simulink model "couche_0"  (R2019b)
settings: Solver=ode23t  StartTime=0.0  StopTime=50  RelTol=1e-3
InitFcn:
  | S = 80   % m2
  | e = 30   % cm
  | p = 2500  % kg/m3
  | lamda = 1.65  %  W/(K.m)
  | C = 880  % J/kg/K
  | k_conv = 25   %  W/(m2.K)
libraries: fl_lib x12, nesl_utility x3
settings Model: Creator=Ivan  LastModifiedBy=Ivan

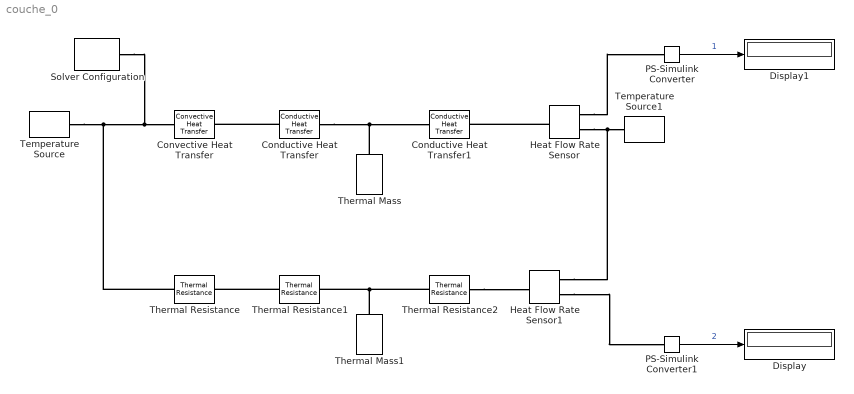
== system couche_0 ==
  Conductive Heat Transfer : fl_lib/Thermal/Thermal Elements/Conductive Heat Transfer  area=S m^2  thickness=e/2 m  th_cond=lamda W/(m*K)  T_specify=off  T_priority=None  T=0 K  T_nominal_specify=off  T_nominal_unit=K  T_nominal_value=1  Q_specify=off  Q_priority=None  Q=0 W  Q_nominal_specify=off  Q_nominal_unit=W  Q_nominal_value=1
      settings: SourceProductName=Simscape
  Conductive Heat Transfer1 : fl_lib/Thermal/Thermal Elements/Conductive Heat Transfer  area=S m^2  thickness=e/2 m  th_cond=lamda W/(m*K)  T_specify=off  T_priority=None  T=0 K  T_nominal_specify=off  T_nominal_unit=K  T_nominal_value=1  Q_specify=off  Q_priority=None  Q=0 W  Q_nominal_specify=off  Q_nominal_unit=W  Q_nominal_value=1
      settings: SourceProductName=Simscape
  Convective Heat Transfer : fl_lib/Thermal/Thermal Elements/Convective Heat Transfer  area=S m^2  heat_tr_coeff=k_conv W/(m^2 * K)  T_specify=off  T_priority=None  T=0 K  T_nominal_specify=off  T_nominal_unit=K  T_nominal_value=1  Q_specify=off  Q_priority=None  Q=0 W  Q_nominal_specify=off  Q_nominal_unit=W  Q_nominal_value=1
  Display : Display
  Display1 : Display
  Heat Flow Rate Sensor : fl_lib/Thermal/Thermal Sensors/Heat Flow Rate Sensor
      settings: SourceProductName=Simscape  SourceProductBaseCode=SS
  Heat Flow Rate Sensor1 : fl_lib/Thermal/Thermal Sensors/Heat Flow Rate Sensor
      settings: SourceProductName=Simscape  SourceProductBaseCode=SS
  PS-Simulink Converter : nesl_utility/PS-Simulink Converter  PhysicalDomain=network_engine_domain  SubClassName=ps_output  LeftPortType=input  RightPortType=output  PseudoPeriodic=off  Frequencies=[]  Unit=W  AffineConversion=off
  PS-Simulink Converter1 : nesl_utility/PS-Simulink Converter  PhysicalDomain=network_engine_domain  SubClassName=ps_output  LeftPortType=input  RightPortType=output  PseudoPeriodic=off  Frequencies=[]  Unit=W  AffineConversion=off
  Solver Configuration : nesl_utility/Solver Configuration  PhysicalDomain=network_engine_domain  SubClassName=solver  LeftPortType=input  RightPortType=generic  Tones=[]  Harmonics=[]  SimulateNoise=off  Profile=off  UseLocalSampling=off  EnableSwitchedLinearOptims=on  FrequencyDomain=off  UseCCode=off  RelTol=0.001  AbsTol=1e-06  MinStep=1e-09  ToWorkspace=off  RevertToSquareIcSolve=off  NumHomotopyIterations=100  PhasorMode=off  PhasorModeNumHarmonics=1  DoDC=off  ResidualTolerance=1e-09  UseLocalSolver=off  LocalSolverChoice=NE_BACKWARD_EULER_ADVANCER  LocalSolverSampleTime=0.001  DoFixedCost=off  MaxNonlinIter=3  MaxModeIter=2  LinearAlgebra=auto  EquationFormulation=NE_TIME_EF  DelaysMemoryBudget=1024  AutomaticFiltering=on  FilteringTimeConstant=0.001  PartitionStorageMethod=AS_NEEDED  PartitionMemoryBudget=1024  PartitionMethod=ROBUST
  Temperature Source : fl_lib/Thermal/Thermal Sources/Temperature Source  temperature=20 degC
      settings: SourceProductName=Simscape
  Temperature Source1 : fl_lib/Thermal/Thermal Sources/Temperature Source  temperature=5 degC
      settings: SourceProductName=Simscape
  Thermal Mass : fl_lib/Thermal/Thermal Elements/Thermal Mass  mass=p*S*e kg  sp_heat=C J/kg/K  T_specify=off  T_priority=High  T=300 K  T_nominal_specify=off  T_nominal_unit=K  T_nominal_value=1  Q_specify=off  Q_priority=None  Q=0 W  Q_nominal_specify=off  Q_nominal_unit=W  Q_nominal_value=1
  Thermal Mass1 : fl_lib/Thermal/Thermal Elements/Thermal Mass  mass=p*S*e kg  sp_heat=C J/kg/K  T_specify=off  T_priority=High  T=300 K  T_nominal_specify=off  T_nominal_unit=K  T_nominal_value=1  Q_specify=off  Q_priority=None  Q=0 W  Q_nominal_specify=off  Q_nominal_unit=W  Q_nominal_value=1
  Thermal Resistance : fl_lib/Thermal/Thermal Elements/Thermal Resistance  resistance=1/ (k_conv*S) K/W  T_specify=off  T_priority=None  T=0 K  T_nominal_specify=off  T_nominal_unit=K  T_nominal_value=1  Q_specify=off  Q_priority=None  Q=0 W  Q_nominal_specify=off  Q_nominal_unit=W  Q_nominal_value=1
      settings: SourceProductName=Simscape  SourceProductBaseCode=SS
  Thermal Resistance1 : fl_lib/Thermal/Thermal Elements/Thermal Resistance  resistance=(e/2)/(S*lamda) K/W  T_specify=off  T_priority=None  T=0 K  T_nominal_specify=off  T_nominal_unit=K  T_nominal_value=1  Q_specify=off  Q_priority=None  Q=0 W  Q_nominal_specify=off  Q_nominal_unit=W  Q_nominal_value=1
      settings: SourceProductName=Simscape  SourceProductBaseCode=SS
  Thermal Resistance2 : fl_lib/Thermal/Thermal Elements/Thermal Resistance  resistance=(e/2)/(S*lamda) K/W  T_specify=off  T_priority=None  T=0 K  T_nominal_specify=off  T_nominal_unit=K  T_nominal_value=1  Q_specify=off  Q_priority=None  Q=0 W  Q_nominal_specify=off  Q_nominal_unit=W  Q_nominal_value=1
      settings: SourceProductName=Simscape  SourceProductBaseCode=SS
  wires:
  PS-Simulink Converter/1 -> Display1/1  "1"
  PS-Simulink Converter1/1 -> Display/1  "2"
  connections:
  Conductive Heat Transfer/RConn1 -- Thermal Mass/LConn1 -- Conductive Heat Transfer1/LConn1
  Conductive Heat Transfer/LConn1 -- Convective Heat Transfer/RConn1
  Temperature Source/LConn1 -- Thermal Resistance/LConn1 -- Solver Configuration/RConn1 -- Convective Heat Transfer/LConn1
  Heat Flow Rate Sensor/LConn1 -- Conductive Heat Transfer1/RConn1
  Heat Flow Rate Sensor/RConn2 -- Heat Flow Rate Sensor1/RConn2 -- Temperature Source1/LConn1
  Heat Flow Rate Sensor/RConn1 -- PS-Simulink Converter/LConn1
  Thermal Mass1/LConn1 -- Thermal Resistance2/LConn1 -- Thermal Resistance1/RConn1
  Heat Flow Rate Sensor1/RConn1 -- PS-Simulink Converter1/LConn1
  Thermal Resistance2/RConn1 -- Heat Flow Rate Sensor1/LConn1
  Thermal Resistance1/LConn1 -- Thermal Resistance/RConn1
